simulink model "EFRP_nl"  (R2020a)
settings: Solver=FixedStepAuto  StartTime=0.0  StopTime=time  FixedStep=0.05  RelTol=1e-5
InitFcn:
  | variableCalc
undefined symbols (not defined in the file): aD1, bd, cd, d0, dd, FOss, GOss, oss0, S, wD1, x0
settings Model: Creator=alfystar  LastModifiedBy=emanu

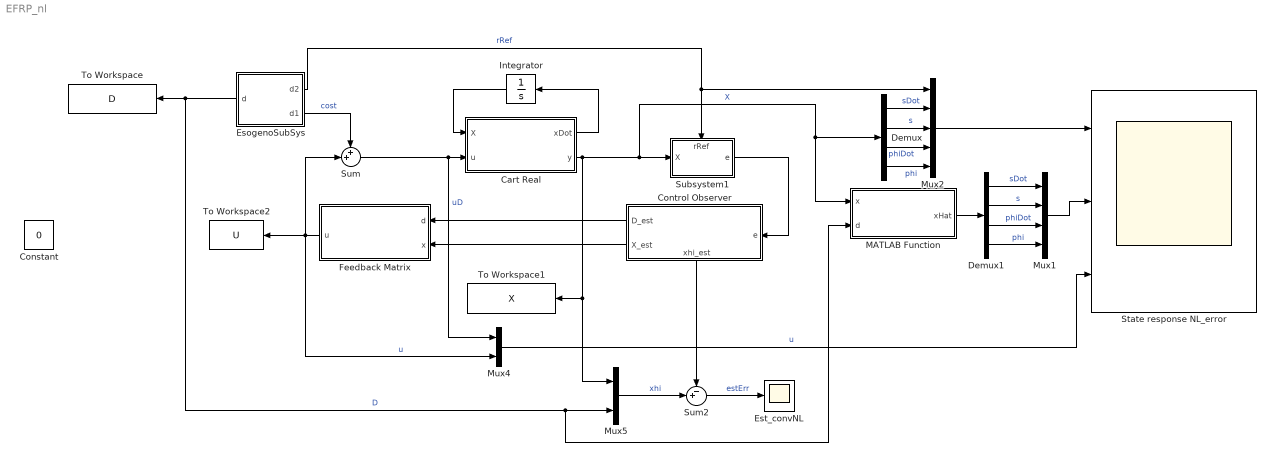
== system EFRP_nl ==
  Cart Real : MATLAB Function  TreatAsAtomicUnit=on
  Constant : Constant  Value=0
  Control Observer : Subsystem
      settings: PortSchema="{\"entries\":[{\"content\":{\"sides\":[{\"content\":{\"connectorIds\":[\"In1\"]},\"type\":\"ConnectorPlacement.EquallySpacedRectSide\",\"uuid\":\"06f85cea-79fe-4a26-b9da-f6471bf8bf3e\"},{\"content\":{\"connectorIds\":[\"Out1\",\"Out2\"],\"side\":\"RIGHT\"},\"type\":\"ConnectorPlacement.EquallySpacedRectSide\",\"uuid\":\"d648b2f6-c54a-4107-ac52-849760b06714\"},{\"content\":{\"connectorIds\":[],\"side\":\"TOP\"},\"type\":\"ConnectorPlacement.EquallySpacedRectSide\",\"uuid\":\"0c8f7184-7dd7-4614-a7a3-a11f49daa96c\"},{\"content\":{\"connectorIds\":[\"Out3\"],\"side\":\"BOTTOM\"},\"type\":\"ConnectorPlacement.EquallySpacedRectSide\",\"uuid\":\"24f6bcc9-5f40-4380-a6f1-f1784c03e5b1\"}]},\"type\":\"ConnectorPlacement.EquallySpacedConnector\",\"uuid\":\"174da35b-9b84-4ac3-b5ca-821bd5eb9ec8\"}],\"packageUris\":[\"http://schema.mathworks.com/mf0/Connector/19700101\"],\"version\":\"1.0\"}"
  Demux : Demux
  Demux1 : Demux
  EsogenoSubSys : Subsystem
      settings: PortSchema="{\"entries\":[{\"content\":{\"sides\":[{\"content\":{\"connectorIds\":[\"Out3\"]},\"type\":\"ConnectorPlacement.EquallySpacedRectSide\",\"uuid\":\"2f048b8f-2ece-4481-a059-706f1c660597\"},{\"content\":{\"connectorIds\":[\"Out1\",\"Out2\"],\"side\":\"RIGHT\"},\"type\":\"ConnectorPlacement.EquallySpacedRectSide\",\"uuid\":\"5f2d4447-8f06-4961-a5d4-88bfa1a982d6\"},{\"content\":{\"connectorIds\":[],\"side\":\"TOP\"},\"type\":\"ConnectorPlacement.EquallySpacedRectSide\",\"uuid\":\"01607c17-a512-406e-96e4-6df13fd083f1\"}]},\"type\":\"ConnectorPlacement.EquallySpacedConnector\",\"uuid\":\"68a4d915-b1c1-450a-8606-a9ee066c43ba\"}],\"packageUris\":[\"http://schema.mathworks.com/mf0/Connector/19700101\"],\"version\":\"1.0\"}"
  Est_convNL : Scope
  Feedback Matrix : MATLAB Function  TreatAsAtomicUnit=on
  Integrator : Integrator  InitialCondition=x0
  MATLAB Function : MATLAB Function  TreatAsAtomicUnit=on
  Mux1 : Mux
  Mux2 : Mux  Inputs=5
  Mux4 : Mux  Inputs=2
  Mux5 : Mux  Inputs=2
  State response NL_error : Scope  NumInputPorts=3
  Subsystem1 : Subsystem
      settings: PortSchema="{\"entries\":[{\"content\":{\"sides\":[{\"content\":{\"connectorIds\":[\"In1\"]},\"type\":\"ConnectorPlacement.EquallySpacedRectSide\",\"uuid\":\"26d6d4a6-782a-4ec1-8ad1-624a6e3a6605\"},{\"content\":{\"connectorIds\":[\"Out1\"],\"side\":\"RIGHT\"},\"type\":\"ConnectorPlacement.EquallySpacedRectSide\",\"uuid\":\"9f19e00a-24c8-46ea-a664-70386d003256\"},{\"content\":{\"connectorIds\":[\"In2\"],\"side\":\"TOP\"},\"type\":\"ConnectorPlacement.EquallySpacedRectSide\",\"uuid\":\"681649f3-5b2c-4efc-a421-7ada1d623381\"}]},\"type\":\"ConnectorPlacement.EquallySpacedConnector\",\"uuid\":\"8cb98563-efc1-437c-a719-f775b8d67a15\"}],\"packageUris\":[\"http://schema.mathworks.com/mf0/Connector/19700101\"],\"version\":\"1.0\"}"
  Sum : Sum  Inputs=++|
  Sum2 : Sum  Inputs=-+|
  To Workspace : ToWorkspace  VariableName=D  SaveFormat=Timeseries  SampleTime=-1
  To Workspace1 : ToWorkspace  VariableName=X  SaveFormat=Timeseries  SampleTime=-1
  To Workspace2 : ToWorkspace  VariableName=U  SaveFormat=Timeseries  SampleTime=-1
  wires:
  Demux/3 -> Mux2/4  "phiDot"
  Demux/4 -> Mux2/5  "phi"
  Mux2/1 -> State response NL_error/1
  Demux/1 -> Mux2/2  "sDot"
  Demux/2 -> Mux2/3  "s"
  Sum/1 -> Cart Real/2(u), Mux4/1  "uD"
  EsogenoSubSys/2(d1) -> Sum/1  "cost"
  Demux1/3 -> Mux1/3  "phiDot"
  Demux1/4 -> Mux1/4  "phi"
  Demux1/2 -> Mux1/2  "s"
  MATLAB Function/1(xHat) -> Demux1/1
  Demux1/1 -> Mux1/1  "sDot"
  Mux1/1 -> State response NL_error/2
  Mux4/1 -> State response NL_error/3  "u"
  Cart Real/2(y) -> Mux5/1, To Workspace1/1, Subsystem1/1(X), MATLAB Function/1(x), Demux/1  "X"
  EsogenoSubSys/1(d2) -> Mux2/1, Subsystem1/2(rRef)  "rRef"
  EsogenoSubSys/3(d) -> To Workspace/1, MATLAB Function/2(d), Mux5/2  "D"
  Feedback Matrix/1(u) -> Sum/2, Mux4/2, To Workspace2/1  "u"
  Mux5/1 -> Sum2/2  "xhi"
  Sum2/1 -> Est_convNL/1  "estErr"
  Subsystem1/1(e) -> Control Observer/1(e)
  Control Observer/1(D_est) -> Feedback Matrix/1(d)
  Control Observer/2(X_est) -> Feedback Matrix/2(x)
  Control Observer/3(xhi_est) -> Sum2/1
  Cart Real/1(xDot) -> Integrator/1
  Integrator/1 -> Cart Real/1(X)

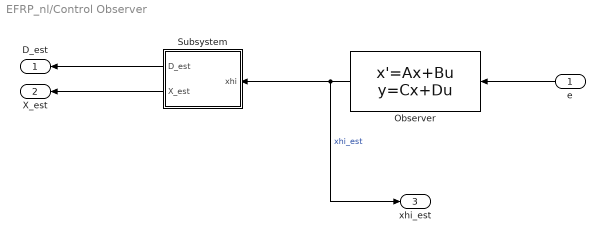
== system EFRP_nl/Control Observer ==
  e : Inport
  Observer : StateSpace  A=FOss  B=GOss  C=eye(7)  D=zeros(7,2)  InitialCondition=oss0
  Subsystem : Subsystem
  D_est : Outport
  X_est : Outport  Port=2
  xhi_est : Outport  Port=3
  wires:
  Subsystem/2(X_est) -> X_est/1
  Observer/1 -> Subsystem/1(xhi), xhi_est/1  "xhi_est"
  Subsystem/1(D_est) -> D_est/1
  e/1 -> Observer/1

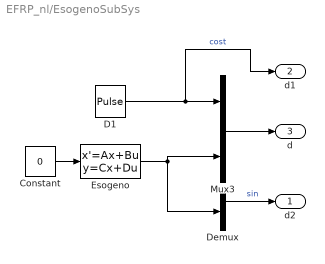
== system EFRP_nl/EsogenoSubSys ==
  Constant : Constant  Value=0
  D1 : DiscretePulseGenerator  PulseType=Time based  Amplitude=aD1  Period=1/wD1  PulseWidth=50
  Demux : Demux  Outputs=2
  Esogeno : StateSpace  A=S  B=bd  C=cd  D=dd  InitialCondition=d0
  Mux3 : Mux  Inputs=2
  d2 : Outport
  d1 : Outport  Port=2
  d : Outport  Port=3
  wires:
  D1/1 -> d1/1, Mux3/1  "cost"
  Esogeno/1 -> Mux3/2, Demux/1
  Constant/1 -> Esogeno/1
  Mux3/1 -> d/1
  Demux/1 -> d2/1  "sin"

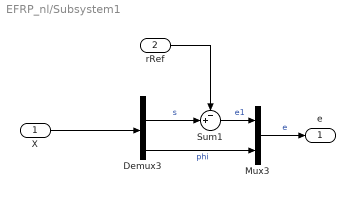
== system EFRP_nl/Subsystem1 ==
  X : Inport
  rRef : Inport  Port=2
  Demux3 : Demux
  Mux3 : Mux  Inputs=2
  Sum1 : Sum  Inputs=-+|
  e : Outport
  wires:
  Mux3/1 -> e/1  "e"
  Demux3/2 -> Sum1/2  "s"
  Sum1/1 -> Mux3/1  "e1"
  X/1 -> Demux3/1
  Demux3/4 -> Mux3/2  "phi"
  rRef/1 -> Sum1/1

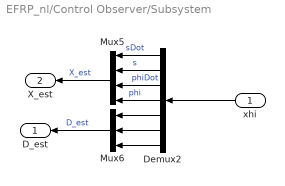
== system EFRP_nl/Control Observer/Subsystem ==
  xhi : Inport
  Demux2 : Demux  Outputs=7
  Mux5 : Mux
  Mux6 : Mux  Inputs=3
  D_est : Outport
  X_est : Outport  Port=2
  wires:
  Demux2/6 -> Mux6/2
  Demux2/2 -> Mux5/2  "s"
  Mux6/1 -> D_est/1  "D_est"
  Demux2/3 -> Mux5/3  "phiDot"
  Demux2/4 -> Mux5/4  "phi"
  Demux2/5 -> Mux6/1
  Demux2/7 -> Mux6/3
  Mux5/1 -> X_est/1  "X_est"
  Demux2/1 -> Mux5/1  "sDot"
  xhi/1 -> Demux2/1

== matlab function EFRP_nl/MATLAB Function ==
  data: x input; xHat output; d input
function xHat = baseChange(x,d)

coder.extrinsic('evalin', 'assignin')
PiMat = zeros(4,3);                  % Needed in order to set variable class correctly
PiMat = evalin('base','PiMat'); % Read value from workspace


xHat = x-PiMat*d;
end

== matlab function EFRP_nl/Feedback Matrix ==
  data: d input; x input; u output
function u = feedMatrix(d,x)

coder.extrinsic('evalin', 'assignin')
K = zeros(1,4);                  % Needed in order to set variable class correctly
K = evalin('base','K'); % Read value from workspace

L = zeros(1,3);                  % Needed in order to set variable class correctly
L = evalin('base','L'); % Read value from workspace

% x(2)=x(2)-d(2);
u=0;
u=K*x+L*d;
end

== matlab function EFRP_nl/Cart Real ==
  data: xDot output; X input; u input; y output
function [xDot,y] = CartSis(X,u)

coder.extrinsic('evalin', 'assignin')
l=1;
l = evalin('base','l'); % Read value from workspace

M=1;
M = evalin('base','M'); % Read value from workspace

F=1;
F = evalin('base','F'); % Read value from workspace

g=9.81;
g = evalin('base','g'); % Read value from workspace

y=X;

xDot=zeros(4,1);
xDot(1) = (u - F*X(1))/M;
xDot(2) = X(1);
xDot(3) = g/l*sin(X(4))+(xDot(1)/l)*cos(X(4));
xDot(4) = X(3);


end
